simulink model "bengji"  (R2023b)
settings: Solver=VariableStepAuto  StartTime=0.0  StopTime=100  RelTol=1e-3
settings Model: Creator=asus  LastModifiedBy=asus

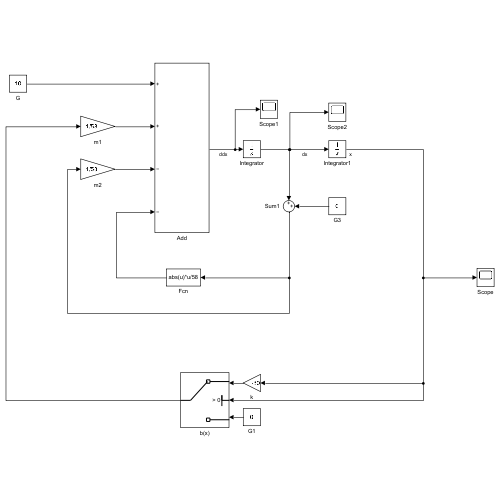
[thumbnail: Simulink's stored preview of the top-level diagram]
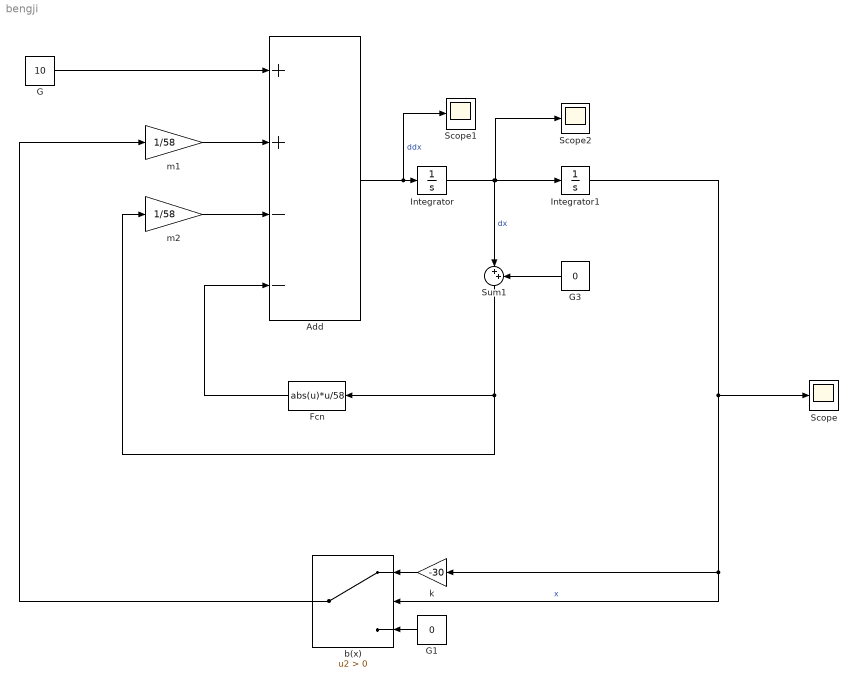
== system bengji ==
  Add : Sum  Inputs=++--
  Fcn : Fcn  Expr=abs(u)*u/58
  G : Constant  Value=10
  G1 : Constant  Value=0
  G3 : Constant  Value=0
  Integrator : Integrator
  Integrator1 : Integrator  InitialCondition=-30
  Scope : Scope
  Scope1 : Scope
  Scope2 : Scope
  Sum1 : Sum  Inputs=|++
  b(x) : Switch  Criteria=u2 > Threshold  SaturateOnIntegerOverflow=off  InputSameDT=off
  k : Gain  Gain=-30
  m1 : Gain  Gain=1/58
  m2 : Gain  Gain=1/58
  wires:
  Add/1 -> Scope1/1, Integrator/1  "ddx"
  G/1 -> Add/1
  b(x)/1 -> m1/1
  G1/1 -> b(x)/3
  k/1 -> b(x)/1
  Integrator/1 -> Integrator1/1, Scope2/1, Sum1/1  "dx"
  m1/1 -> Add/2
  m2/1 -> Add/3
  Fcn/1 -> Add/4
  Integrator1/1 -> Scope/1, b(x)/2, k/1  "x"
  Sum1/1 -> m2/1, Fcn/1
  G3/1 -> Sum1/2
